simulink model "arduinomega2560_communication"  (Simulink 10.0)
settings: Solver=ode3  StartTime=0.0  StopTime=inf  RelTol=1e-3
libraries: arduinolib x1, simulink x1
PreSaveFcn:
  | set_param(gcs, 'location', [45 95 785 420])
settings Model: FPTRunName=Active  Creator=The MathWorks Inc.  LastModifiedBy=bhisma  ExtModeTrigDuration=2
settings DataIOCC: LimitDataPoints=on  SignalLoggingSaveFormat=ModelDataLogs
settings OptimizationCC: ExpressionDepthLimit=2147483647  LifeSpan=Inf  EfficientTunableParamExpr=on
settings DebuggingCC: FcnCallInpInsideContextMsg=warning  StateNameClashWarn=warning
settings HardwareCC: ProdBitPerInt=16  ProdBitPerPointer=16  ProdBitPerSizeT=16  ProdBitPerPtrDiffT=16  ProdIntDivRoundTo=Zero  ProdEndianess=LittleEndian  ProdWordSize=8  ProdHWDeviceType=Atmel->AVR
settings SFSimCC: MATLABDynamicMemAlloc=off
settings RTWCC: Description=Real-Time Toolbox  SystemTargetFile=realtime.tlc  GenerateMakefile=off  TemplateMakefile=realtime.tmf  RTWVerbose=off
settings CodeAppCC: CustomSymbolStrType=$N$R$M  InternalIdentifier=Classic
settings STFCustomTargetCC: TargetLibSuffix=.a  GenerateSampleERTMain=on  ERTCustomFileBanners=on  SupportNonInlinedSFcns=off  RemoveResetFunc=on  SupportVariableSizeSignals=on  MATLABClassNameForMDSCustomization=Simulink.SoftwareTarget.ERTCustomization  GRTInterface=off  SystemTargetFile=realtime.tlc
settings ERTTargetCC: MultiwordLength=2048  GenerateSampleERTMain=on  ParMdlRefBuildCompliant=off  CompOptLevelCompliant=off  ConcurrentExecutionCompliant=off  CombineOutputUpdateFcns=off  SupportContinuousTime=on  SupportVariableSizeSignals=on  ModelStepFunctionPrototypeControlCompliant=off  CPPClassGenCompliant=off  UseToolchainInfoCompliant=off  ExtModeTransport=3  ExtModeMexFile=ext_serial_win32_comm  ExtModeMexArgs=0 1 115200  ERTSrcFileBannerTemplate=realtime_code_template.cgt  ERTHdrFileBannerTemplate=realtime_code_template.cgt  ERTDataSrcFileTemplate=realtime_code_template.cgt  ERTDataHdrFileTemplate=realtime_code_template.cgt  ERTCustomFileTemplate=realtime_file_process.tlc  ConvertIfToSwitch=off  SuppressUnreachableDefaultCases=off
settings ConfigComp: CovExternalEMLEnable=off
settings SettingsController: Description=Run on Hardware Dialog  TargetExtensionPlatform=Arduino Mega 2560
settings MATStruct: Set_host_COM_port=[0.0]  COM_port_number=1  COM_port_baud_rate=115200  Enable_overrun_detection=[0.0]  Digital_output_to_set_on_overrun=13  Analog_input_reference_voltage=[0.0]  Serial1_baud_rate=9600  Serial2_baud_rate=9600  Serial3_baud_rate=9600  Serial0_baud_rate=115200

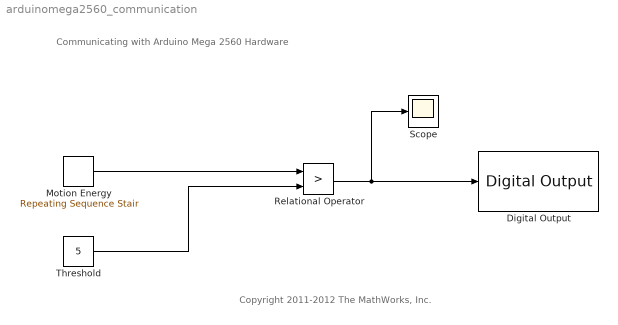
== system arduinomega2560_communication ==
  note: Communicating with Arduino Mega 2560 Hardware
  note: Copyright 2011-2012 The MathWorks, Inc.
  Digital Output : arduinolib/Digital Output  pinNumber=9
  Motion Energy : simulink/Sources/Repeating Sequence Stair  OutValues=|  tsamp=0.1  OutMin=[]  OutMax=[]  OutDataTypeStr=uint8  OutputDataTypeScalingMode=uint8  OutDataType=fixdt(0,8)  ConRadixGroup=Best Precision: Vector-wise  OutScaling=2^-12
      | [ 3
      |     2
      |     2
      |     1
      |     1
      |     1
      |     1
      |     1
      |     1
      |     1
      |     1
      |     1
      |     1
      |     2
      |     3
      |     3
      |     4
      |     4
      |     5
      |     5
      |     5
      |     6
      |     5
      |     6
      |     6
      |     6
      |     7
      |     8
      |     8
      |     8
      |     9
      |     9
      |     9
      |     9
      |     9
      |    10
      |    12
      |    12
      |    11
      |    10
      |    10
      |     9
      |     8
      |     7
      |     5
      |     6
      |     5
      |     4
      |     4
      |     5
      |     5
      |     4
      |     4
      |     4
      |     3
      |     3
      |     2
      |     2
      |     2
      |     2
      |     2
      |     2
      |     2
      |     2
      |     2
      |     2
      |     1
      |     1
      |     2
      |     2
      |     2
      |     1
      |     2
      |     2
      |     2
      |     2
      |     2
      |     2
      |     2
      |     2
      |     2
      |     2
      |     2
      |     3
      |     2
      |     2
      |     3
      |     3
      |     3
      |     4
      |     4
      |     4
      |     4
      |     4
      |     4
      |     4
      |     4
      |     4
      |     4
      |     7
      |     4
      |     42
      |    39
      |     46
      |     6
      |     6
      |     7
      |     6
      |     6
      |     5
      |     5
      |     4
      |     4
      |     5
      |     5
      |     6
      |    53
      |     47
      |     50
      |     5
      |     5
      |     5
      |     6
      |     7
      |     8
      |     7
      |     7
      |     6
      |     6
      |     7
      |     8
      |     9
      |    19
      |     8
      |     8
      |     6
      |     6
      |     5
      |     5
      |     5
      |     4
      |     4
      |     4
      |     4
      |     4
      |     5
      |    17
      |     5
      |     4
      |     4]'
  Relational Operator : RelationalOperator  Operator=>  OutDataTypeStr=fixdt(1,16)  RndMeth=Nearest
  Scope : Scope
  "Threshold " : Constant  Value=5  OutDataTypeStr=uint8  SampleTime=0.1
  wires:
  Motion Energy/1 -> Relational Operator/1
  Relational Operator/1 -> Scope/1, Digital Output/1
  "Threshold "/1 -> Relational Operator/2
